simulink model "inga"  (R2021a)
settings: Solver=VariableStepAuto  StartTime=0.0  StopTime=500  RelTol=1e-3
settings Model: Creator=Krisz  LastModifiedBy=Krisz

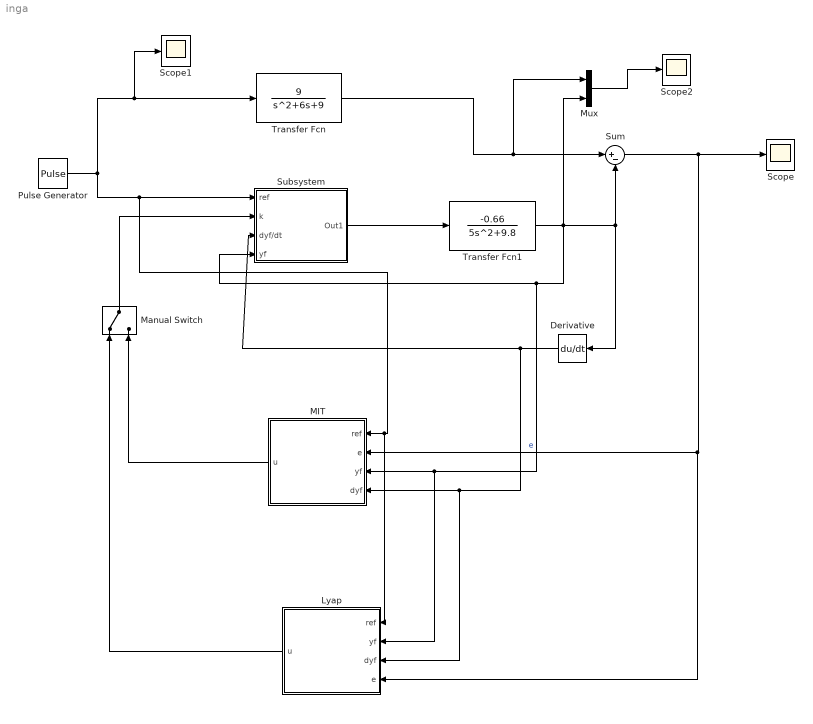
== system inga ==
  Derivative : Derivative
  Lyap : Subsystem
  MIT : Subsystem
  Manual Switch : ManualSwitch
  Mux : Mux  Inputs=2
  Pulse Generator : DiscretePulseGenerator  PulseType=Time based  Amplitude=5  Period=50  PulseWidth=50
  Scope : Scope
  Scope1 : Scope
  Scope2 : Scope
  Subsystem : Subsystem
  Sum : Sum  Inputs=|+-
  Transfer Fcn : TransferFcn  Numerator=[9]  Denominator=[1 6 9]
  Transfer Fcn1 : TransferFcn  Numerator=[-0.66]  Denominator=[5 0 9.8]
  wires:
  Transfer Fcn1/1 -> Mux/2, Lyap/2(yf), MIT/3(yf), Subsystem/4(yf), Sum/2, Derivative/1
  Transfer Fcn/1 -> Mux/1, Sum/1
  Subsystem/1(Out1) -> Transfer Fcn1/1
  Pulse Generator/1 -> Lyap/1(ref), MIT/1(ref), Subsystem/1(ref), Scope1/1, Transfer Fcn/1
  Sum/1 -> Lyap/4(e), MIT/2(e), Scope/1  "e"
  Derivative/1 -> Lyap/3(dyf), MIT/4(dyf), Subsystem/3(dyf/dt)
  Manual Switch/1 -> Subsystem/2(k)
  MIT/1(u) -> Manual Switch/2
  Mux/1 -> Scope2/1
  Lyap/1(u) -> Manual Switch/1

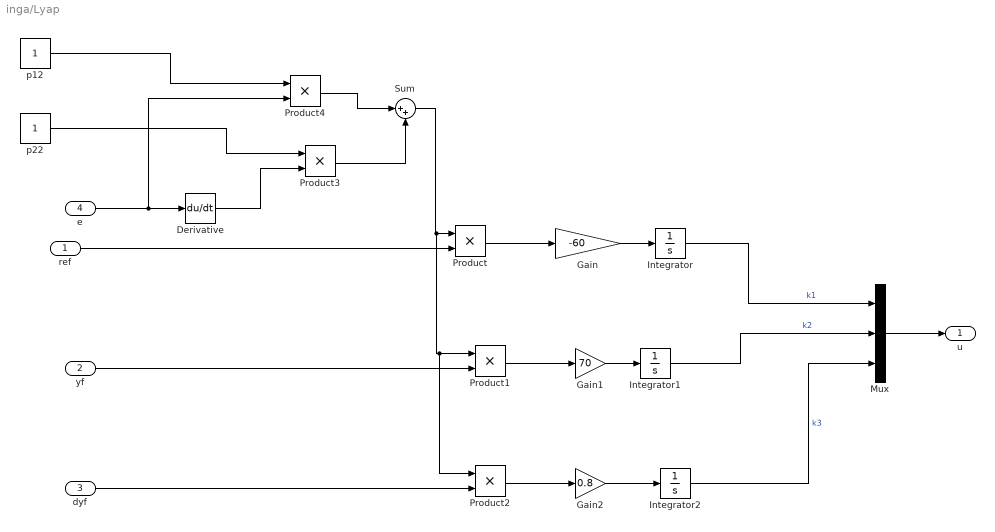
== system inga/Lyap ==
  ref : Inport
  yf : Inport  Port=2
  dyf : Inport  Port=3
  e : Inport  Port=4
  Derivative : Derivative
  Gain : Gain  Gain=-60
  Gain1 : Gain  Gain=70
  Gain2 : Gain  Gain=0.8
  Integrator : Integrator
  Integrator1 : Integrator
  Integrator2 : Integrator
  Mux : Mux  Inputs=3
  Product{,1..4} (5 alike) : Product
  Sum : Sum  Inputs=|++
  p12 : Constant
  p22 : Constant
  u : Outport
  wires:
  Mux/1 -> u/1
  Product2/1 -> Gain2/1
  Product1/1 -> Gain1/1
  Product/1 -> Gain/1
  Gain/1 -> Integrator/1
  Gain1/1 -> Integrator1/1
  Gain2/1 -> Integrator2/1
  yf/1 -> Product1/2
  dyf/1 -> Product2/2
  Integrator/1 -> Mux/1  "k1"
  Integrator1/1 -> Mux/2  "k2"
  Integrator2/1 -> Mux/3  "k3"
  ref/1 -> Product/2
  Derivative/1 -> Product3/2
  Product3/1 -> Sum/2
  Sum/1 -> Product2/1, Product1/1, Product/1
  e/1 -> Product4/2, Derivative/1
  Product4/1 -> Sum/1
  p12/1 -> Product4/1
  p22/1 -> Product3/1

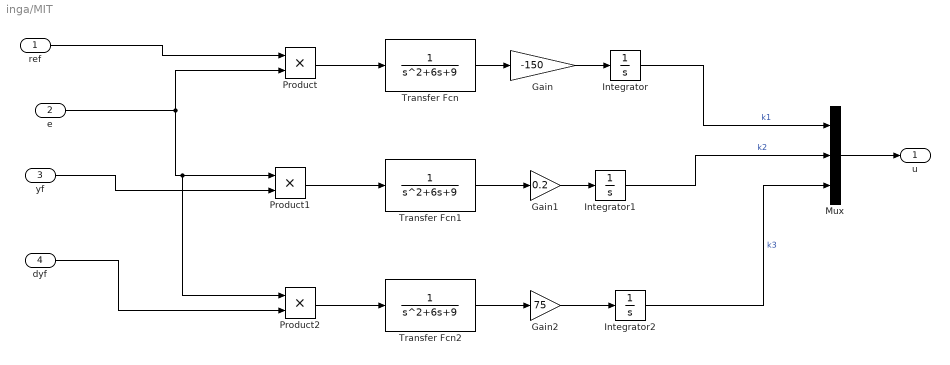
== system inga/MIT ==
  ref : Inport
  e : Inport  Port=2
  yf : Inport  Port=3
  dyf : Inport  Port=4
  Gain : Gain  Gain=-150
  Gain1 : Gain  Gain=0.2
  Gain2 : Gain  Gain=75
  Integrator : Integrator
  Integrator1 : Integrator
  Integrator2 : Integrator
  Mux : Mux  Inputs=3
  Product : Product
  Product1 : Product
  Product2 : Product
  Transfer Fcn : TransferFcn  Denominator=[1 6 9]
  Transfer Fcn1 : TransferFcn  Denominator=[1 6 9]
  Transfer Fcn2 : TransferFcn  Denominator=[1 6 9]
  u : Outport
  wires:
  Product/1 -> Transfer Fcn/1
  Product1/1 -> Transfer Fcn1/1
  ref/1 -> Product/1
  e/1 -> Product2/1, Product1/1, Product/2
  Mux/1 -> u/1
  Product2/1 -> Transfer Fcn2/1
  Transfer Fcn2/1 -> Gain2/1
  Transfer Fcn1/1 -> Gain1/1
  Transfer Fcn/1 -> Gain/1
  Gain/1 -> Integrator/1
  Gain1/1 -> Integrator1/1
  Gain2/1 -> Integrator2/1
  yf/1 -> Product1/2
  dyf/1 -> Product2/2
  Integrator/1 -> Mux/1  "k1"
  Integrator1/1 -> Mux/2  "k2"
  Integrator2/1 -> Mux/3  "k3"

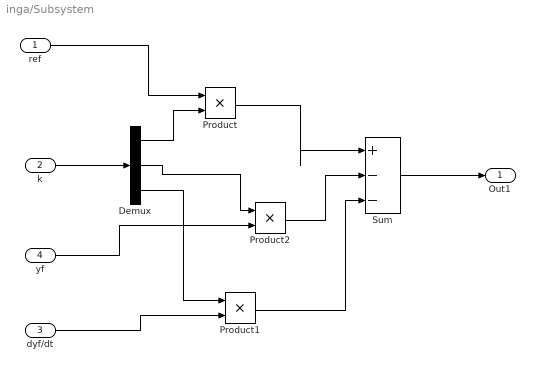
== system inga/Subsystem ==
  ref : Inport
  k : Inport  Port=2
  dyf/dt : Inport  Port=3
  yf : Inport  Port=4
  Demux : Demux  Outputs=3
  Product : Product
  Product1 : Product
  Product2 : Product
  Sum : Sum  Inputs=|+--
  Out1 : Outport
  wires:
  ref/1 -> Product/1
  k/1 -> Demux/1
  Demux/1 -> Product/2
  dyf/dt/1 -> Product1/2
  Demux/3 -> Product1/1
  yf/1 -> Product2/2
  Demux/2 -> Product2/1
  Product/1 -> Sum/1
  Product2/1 -> Sum/2
  Product1/1 -> Sum/3
  Sum/1 -> Out1/1
